simulink model "LuenbergerNonLinear"  (R2019a)
settings: Solver=VariableStepAuto  StartTime=0.0  StopTime=40  RelTol=1e-3
values from neighbouring files (symbols this model uses):
  A_OBXT12 = [ 0, 1,         0, 0,        0, 0 ... (first row only)    [LuenbergerObsvXT12.m]
  B_OBXT12 = [0 ... (first row only)    [LuenbergerObsvXT12.m]
  CT12 = [1 0 0 0 0 0 ... (first row only)    [LuenbergerObsvXT12.m]    (also in ObservabilityCheck.m = [0 0 0 0 0 0)
libraries: eeLuenbergerObserver x1
settings Model: Creator=Prasheel Renkuntla  LastModifiedBy=Prasheel Renkuntla

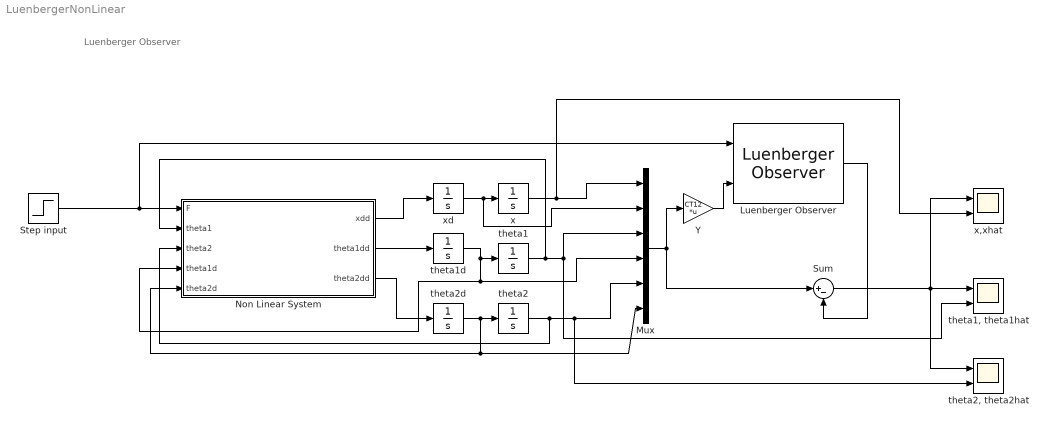
== system LuenbergerNonLinear ==
  note: Luenberger Observer
  Luenberger Observer : eeLuenbergerObserver/Luenberger Observer  StateSpaceType=Continuous-time  Ad=1  Bd=1  Cd=1  Dd=1  A=A_OBXT12  B=B_OBXT12  C=CT12  D=[0;0;0]  ObserverDesign=Desired eigenvalues  Ld=1  DesiredEigenvalues=[-0.1 -0.2 -0.3 -0.4 -0.5 -0.6]  x0=[3; 0; 0.5; 0; 0.5; 0]  Tsd=0.1  Ts=0.1
      settings: SourceProductName=Simscape Electrical  SourceProductBaseCode=PS
  Mux : Mux  Inputs=6
  "Non Linear System " : MATLAB Function  TreatAsAtomicUnit=on
  Step input : Step  SampleTime=0
  Sum : Sum  Inputs=|+-
  Y : Gain  Gain=CT12  Multiplication=Matrix(K*u)
  theta1 : Integrator
  "theta1, theta1hat" : Scope  NumInputPorts=2
  theta1d : Integrator
  theta2 : Integrator
  "theta2, theta2hat" : Scope  NumInputPorts=2
  theta2d : Integrator
  x : Integrator
  x,xhat : Scope  NumInputPorts=2
  xd : Integrator
  wires:
  "Non Linear System "/3(theta2dd) -> theta2d/1
  Mux/1 -> Sum/1, Y/1
  "Non Linear System "/2(theta1dd) -> theta1d/1
  theta2d/1 -> "Non Linear System "/5(theta2d), Mux/6, theta2/1
  theta2/1 -> "Non Linear System "/3(theta2), "theta2, theta2hat"/2, Mux/5
  "Non Linear System "/1(xdd) -> xd/1
  x/1 -> x,xhat/2, Mux/1
  theta1d/1 -> "Non Linear System "/4(theta1d), Mux/4, theta1/1
  theta1/1 -> "Non Linear System "/2(theta1), "theta1, theta1hat"/2, Mux/3
  Step input/1 -> Luenberger Observer/1, "Non Linear System "/1(F)
  xd/1 -> Mux/2, x/1
  Y/1 -> Luenberger Observer/2
  Sum/1 -> x,xhat/1, "theta1, theta1hat"/1, "theta2, theta2hat"/1
  Luenberger Observer/1 -> Sum/2

== matlab function LuenbergerNonLinear/Non Linear System  ==
  data: F input; xdd output; theta1 input; theta2 input; theta1d input; theta2d input; theta1dd output; theta2dd output
function [xdd, theta1dd, theta2dd] = NL(F, theta1, theta2, theta1d, theta2d)
M = 1000;
m1 = 100;
m2 = 100;
l1 = 20;
l2 = 10;
g =9.8;
xdd = (F - m1*g*sind(theta1)*cosd(theta1) - m2*g*sind(theta2)*cosd(theta2) - m1*l1*theta1d*theta1d*sind(theta1) - m2*l2*theta2d*theta2d*sind(theta2))/(M + m1*sind(theta1)*sind(theta1) + m2*sind(theta2)*sind(theta2));
theta1dd = (xdd*cosd(theta1) - g*(sind(theta1)))/(l1);
theta2dd = (xdd*cosd(theta2) - g*(sind(theta2)))/(l2);
end
